simulink model "sgMdl_IO204_DigitalLoopback"  (R2024b)
settings: Solver=FixedStepAuto  StartTime=0.0  StopTime=inf  RelTol=1e-3  EnableMultiTasking=on
libraries: speedgoatlib_IO204 x3
Description:
  | IO204 - Digital Loopback
settings Model: ModifiedByFormat=Speedgoat  Creator=Speedgoat  LastModifiedBy=Speedgoat
settings SolverCC: ConcurrentTasks=on  AlgebraicLoopSolver=TrustRegion  PositivePriorityOrder=on
settings DataIOCC: LimitDataPoints=on  SaveFormat=Array  SignalLoggingSaveFormat=ModelDataLogs  ReturnWorkspaceOutputs=off
settings OptimizationCC: BlockReduction=off  OptimizeBlockIOStorage=off  BufferReuse=off  ReuseModelBlockBuffer=off  GlobalBufferReuse=off  ExpressionFolding=off  ExpressionDepthLimit=2147483647  LocalBlockOutputs=off
settings DebuggingCC: UnderspecifiedInitializationDetection=Classic  MergeDetectMultiDrivingBlocksExec=none  SolverPrmCheckMsg=warning  TasksWithSamePriorityMsg=none  FcnCallInpInsideContextMsg=warning  StateNameClashWarn=warning  SFUnexpectedBacktrackingDiag=warning  SFNoUnconditionalDefaultTransitionDiag=warning  SFExecutionAtInitializationDiag=none  ArithmeticOperatorsInVariantConditions=warning
settings HardwareCC: ProdBitPerLong=64  ProdLongLongMode=on  ProdHWDeviceType=Intel->x86-64 (Linux 64)
settings ModelReferenceCC: EnableRefExpFcnMdlSchedulingChecks=on  PropagateSignalLabelsOutOfModel=off
settings SFSimCC: SimUseLocalCustomCode=off  CustomCodeUndefinedFunction=UseInterfaceOnly
settings RTWCC: Description=Speedgoat Real-Time Target Machine  SystemTargetFile=speedgoat.tlc  TemplateMakefile=slrealtime_default_tmf  RTWUseLocalCustomCode=off  Toolchain=Simulink Real-Time Toolchain  BuildConfiguration=Faster Runs  TargetLang=C++  GPUComputeCapability=3.5  DLArmComputeVersion=19.05
settings CodeAppCC: StateflowObjectComments=on
settings SimulinkRealTimeTargetCC: SubcomponentCodeInterfacePackaging=Reusable function  InstructionSetFMA=off  LogToMDFFile=off  SLRTFileLogMaxRuns=10  UseGCCFastMath=on
settings ConfigComp: CovMetricSettings=dw  CovSaveCumulativeToWorkspaceVar=on  CovSaveSingleToWorkspaceVar=on  CovExternalEMLEnable=off  CovSFcnEnable=off  CovBoundaryAbsTol=1.0e-5

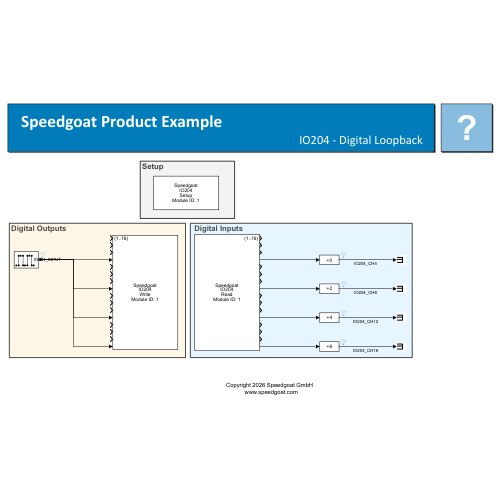
[thumbnail: Simulink's stored preview of the top-level diagram]
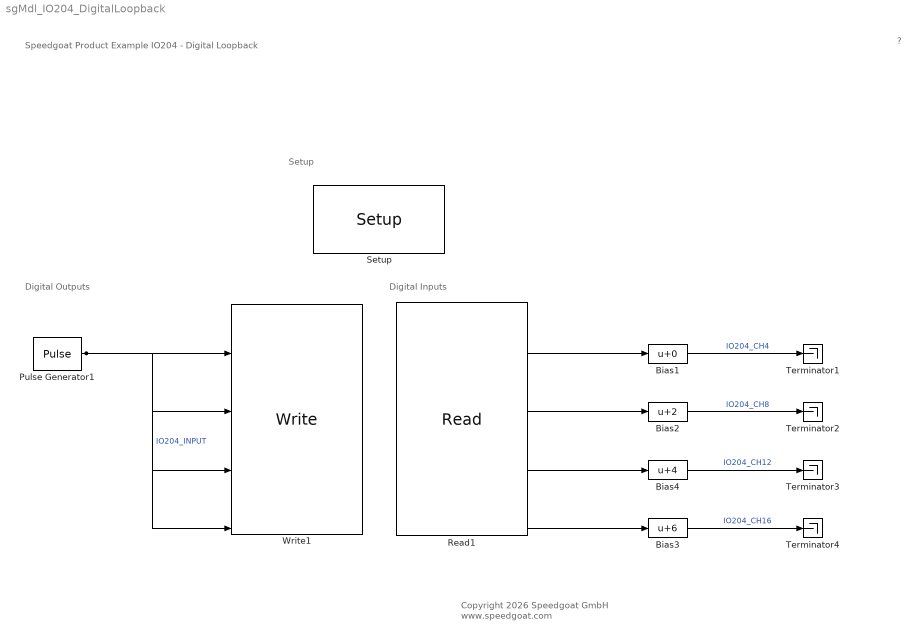
== system sgMdl_IO204_DigitalLoopback ==
  note: Digital Outputs
  note: Digital Inputs
  note: Setup
  note: Speedgoat Product Example
      | IO204 - Digital Loopback
  note: ?
  note: Copyright 2026 Speedgoat GmbH
      |  www.speedgoat.com
  Bias1 : Bias  SaturateOnIntegerOverflow=off
  Bias2 : Bias  Bias=2  SaturateOnIntegerOverflow=off
  Bias3 : Bias  Bias=6  SaturateOnIntegerOverflow=off
  Bias4 : Bias  Bias=4  SaturateOnIntegerOverflow=off
  Pulse Generator1 : DiscretePulseGenerator  Amplitude=0.8  Period=200  PulseWidth=100  SampleTime=0.001
  Read1 : speedgoatlib_IO204/Read  id=1  group=Input  portType=16 ports of type double  ts=0.001  pciSlot=-1
      settings: SourceProductName=Simulink Real-Time: Speedgoat I/O Blockset
  Setup : speedgoatlib_IO204/Setup  group=Module setup  id=1  pciSlot=-1  debounceEnable=on  debounceValue=0.001/10  reset=[0]  value=[0]
      settings: SourceProductName=Simulink Real-Time: Speedgoat I/O Blockset
  Terminator{1..4} (4 alike) : Terminator
  Write1 : speedgoatlib_IO204/Write  id=1  portType=16 ports of type double  ts=-1  pciSlot=-1
      settings: SourceProductName=Simulink Real-Time: Speedgoat I/O Blockset
  wires:
  Bias2/1 -> Terminator2/1  "IO204_CH8"
  Bias1/1 -> Terminator1/1  "IO204_CH4"
  Bias4/1 -> Terminator3/1  "IO204_CH12"
  Bias3/1 -> Terminator4/1  "IO204_CH16"
  Pulse Generator1/1 -> Write1/4, Write1/8, Write1/12, Write1/16  "IO204_INPUT"
  Read1/16 -> Bias3/1
  Read1/12 -> Bias4/1
  Read1/4 -> Bias1/1
  Read1/8 -> Bias2/1
